simulink model "SecRwLtStFwdBkwdIsPosChk"  (R2024b)
settings: Solver=FixedStepDiscrete  StartTime=0.0  StopTime=10.0  FixedStep=0.01  RelTol=1e-3
undefined symbols (not defined in the file or in its folder): KeSMSuSecRwStFwdBkwdPosDelta_Val, KeSMSuSecRwStFwdBkwdPosTolr_Val
libraries: StIsPosChkLib x11, simulink x7
(part 1 of 2)
settings Model: Creator=sn2xws  LastModifiedBy=sn55gm
settings Model: ModifiedHistory=|
  | 2023.8.1 V2.0.0 CR421790 增加模式21-26
  | 2023.9.14 V2.1.0 Bug 540886 修改亲密模式判断到位的条件为10ms周期计算
  | 2023.11.16 V2.3.0 Issue 566045 全躺，vip，腿托打开增加前后位置
  | 2024.7.8 V3.0.0 557模式流程V1.9
  | 2024.8.15 V3.0.1 智享模式需要计算目标位置，不能直接判断到位置，posalready赋值0
  | 2024.9.4 V3.0.2 增加模式Md56，注释不使用的模式
  | 2024.9.18 V3.0.3 Md27 被误注释恢复
  | 2024.10.28 V3.0.4 Md56Calib标签名使用错误导致Md56前后目标位置为0
  | 2024.12.17 V3.0.5 Md57 Md58 报失败问题
  | 25.7.1 V3.13.0 新增Md61Md62
settings SolverCC: AlgebraicLoopSolver=TrustRegion
settings DataIOCC: SaveFormat=StructureWithTime  ReturnWorkspaceOutputs=off
settings OptimizationCC: DefaultParameterBehavior=Inlined  EnhancedBackFolding=on  PassReuseOutputArgsAs=Individual arguments  ZeroExternalMemoryAtStartup=off  ZeroInternalMemoryAtStartup=off  OptimizeBlockOrder=speed  DifferentSizesBufferReuse=on  OptimizationCustomize=off  EfficientTunableParamExpr=on
settings DebuggingCC: ParameterTunabilityLossMsg=error  UnconnectedInputMsg=warning  UnconnectedOutputMsg=warning  UnconnectedLineMsg=warning  ArithmeticOperatorsInVariantConditions=warning
settings ModelReferenceCC: EnableRefExpFcnMdlSchedulingChecks=on  ModelReferenceNumInstancesAllowed=Single
settings SFSimCC: MATLABDynamicMemAlloc=off  CustomCodeUndefinedFunction=UseInterfaceOnly
settings RTWCC: Description=AUTOSAR  SystemTargetFile=autosar.tlc  GenCodeOnly=on  TemplateMakefile=ert_default_tmf  GenerateReport=on  IncludeHyperlinkInReport=on  LaunchReport=on  DataTypeReplacement=CDataTypesFixedWidth  GenerateTraceInfo=on  GenerateTraceReport=on  GenerateTraceReportSl=on  GenerateTraceReportSf=on  GenerateTraceReportEml=on  GenerateCodeMetricsReport=on  GPUComputeCapability=3.5
settings CodeAppCC: ForceParamTrailComments=on  IgnoreCustomStorageClasses=off  OperatorAnnotations=on  SimulinkDataObjDesc=on  SFDataObjDesc=on  InsertBlockDesc=on
settings STFCustomTargetCC: TargetLangStandard=C99 (ISO)  MultiwordLength=256  ParMdlRefBuildCompliant=on  CompOptLevelCompliant=on  IncludeMdlTerminateFcn=off  CombineOutputUpdateFcns=on  SuppressErrorStatus=on  ERTCustomFileBanners=on  SupportNonFinite=off  SupportComplex=off  SupportContinuousTime=off  SupportNonInlinedSFcns=off  RemoveResetFunc=on  MATLABClassNameForMDSCustomization=Simulink.SoftwareTarget.ERTCustomization  AutosarCompliant=on  UseToolchainInfoCompliant=on  LookupTableObjectStructAxisOrder=2,1,3,4,...  LUTObjectStructOrderEvenSpacing=Size,Table,Breakpoints  SystemTargetFile=autosar.tlc
settings ERTTargetCC: TargetLangStandard=C99 (ISO)  ConcurrentExecutionCompliant=off  IncludeMdlTerminateFcn=off  SuppressErrorStatus=on  SupportNonFinite=off  SupportComplex=off  ModelStepFunctionPrototypeControlCompliant=off  CPPClassGenCompliant=off  AutosarCompliant=on  LookupTableObjectStructAxisOrder=2,1,3,4,...  LUTObjectStructOrderEvenSpacing=Size,Table,Breakpoints  ERTCustomFileTemplate=example_file_process.tlc  ERTFilePackagingFormat=Compact  BooleanTrueId=TRUE  BooleanFalseId=FALSE  DynamicArrayContainerType=coder::array

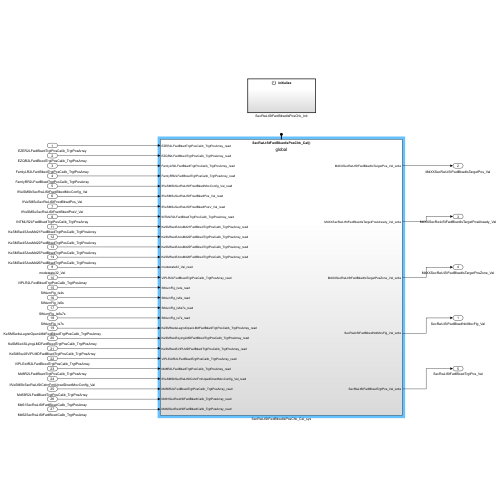
[thumbnail: Simulink's stored preview of the top-level diagram]
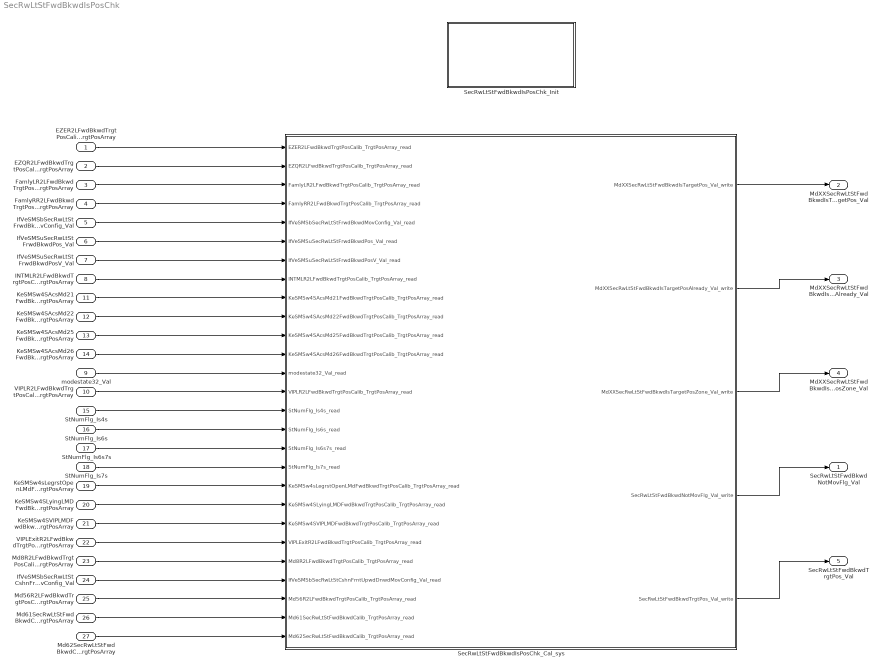
== system SecRwLtStFwdBkwdIsPosChk ==
  EZER2LFwdBkwdTrgtPosCalib_TrgtPosArray : Inport  Description=|  OutDataTypeStr=uint16  PortDimensions=3
      | 0:Pos
      | 1:Max
      | 2:Min
  EZQR2LFwdBkwdTrgtPosCalib_TrgtPosArray : Inport  Description=|  Port=2  OutDataTypeStr=uint16  PortDimensions=3
      | 0:Pos
      | 1:Max
      | 2:Min
  FamlyLR2LFwdBkwdTrgtPosCalib_TrgtPosArray : Inport  Description=|  Port=3  OutDataTypeStr=uint16  PortDimensions=3
      | 0:Pos
      | 1:Max
      | 2:Min
  FamlyRR2LFwdBkwdTrgtPosCalib_TrgtPosArray : Inport  Description=|  Port=4  OutDataTypeStr=uint16  PortDimensions=3
      | 0:Pos
      | 1:Max
      | 2:Min
  IfVeSMSbSecRwLtStFrwdBkwdMovConfig_Val : Inport  Port=5  OutDataTypeStr=boolean  PortDimensions=1
  IfVeSMSuSecRwLtStFrwdBkwdPos_Val : Inport  Port=6  OutDataTypeStr=uint16  PortDimensions=1
  IfVeSMSuSecRwLtStFrwdBkwdPosV_Val : Inport  Port=7  OutDataTypeStr=boolean  PortDimensions=1
  INTMLR2LFwdBkwdTrgtPosCalib_TrgtPosArray : Inport  Description=|  Port=8  OutDataTypeStr=uint16  PortDimensions=3
      | 0:Pos
      | 1:Max
      | 2:Min
  modestate32_Val : Inport  Port=9  OutDataTypeStr=uint32  PortDimensions=1
  VIPLR2LFwdBkwdTrgtPosCalib_TrgtPosArray : Inport  Description=|  Port=10  OutDataTypeStr=uint16  PortDimensions=3
      | 0:Pos
      | 1:Max
      | 2:Min
  KeSMSw4SAcsMd21FwdBkwdTrgtPosCalib_TrgtPosArray : Inport  Description=|  Port=11  OutDataTypeStr=uint16  PortDimensions=3
      | 0:Pos
      | 1:Max
      | 2:Min
  KeSMSw4SAcsMd22FwdBkwdTrgtPosCalib_TrgtPosArray : Inport  Description=|  Port=12  OutDataTypeStr=uint16  PortDimensions=3
      | 0:Pos
      | 1:Max
      | 2:Min
  KeSMSw4SAcsMd25FwdBkwdTrgtPosCalib_TrgtPosArray : Inport  Description=|  Port=13  OutDataTypeStr=uint16  PortDimensions=3
      | 0:Pos
      | 1:Max
      | 2:Min
  KeSMSw4SAcsMd26FwdBkwdTrgtPosCalib_TrgtPosArray : Inport  Description=|  Port=14  OutDataTypeStr=uint16  PortDimensions=3
      | 0:Pos
      | 1:Max
      | 2:Min
  StNumFlg_Is4s : Inport  Port=15  OutDataTypeStr=boolean  PortDimensions=1
  StNumFlg_Is6s : Inport  Port=16  OutDataTypeStr=boolean  PortDimensions=1
  StNumFlg_Is6s7s : Inport  Port=17  OutDataTypeStr=boolean  PortDimensions=1
  StNumFlg_Is7s : Inport  Port=18  OutDataTypeStr=boolean  PortDimensions=1
  KeSMSw4sLegrstOpenLMdFwdBkwdTrgtPosCalib_TrgtPosArray : Inport  Description=|  Port=19  OutDataTypeStr=uint16  PortDimensions=3
      | 0:Pos
      | 1:Max
      | 2:Min
  KeSMSw4SLyingLMDFwdBkwdTrgtPosCalib_TrgtPosArray : Inport  Description=|  Port=20  OutDataTypeStr=uint16  PortDimensions=3
      | 0:Pos
      | 1:Max
      | 2:Min
  KeSMSw4SVIPLMDFwdBkwdTrgtPosCalib_TrgtPosArray : Inport  Description=|  Port=21  OutDataTypeStr=uint16  PortDimensions=3
      | 0:Pos
      | 1:Max
      | 2:Min
  VIPLExitR2LFwdBkwdTrgtPosCalib_TrgtPosArray : Inport  Description=|  Port=22  OutDataTypeStr=uint16  PortDimensions=3
      | 0:Pos
      | 1:Max
      | 2:Min
  Md8R2LFwdBkwdTrgtPosCalib_TrgtPosArray : Inport  Description=|  Port=23  OutDataTypeStr=uint16  PortDimensions=3
      | 0:Pos
      | 1:Max
      | 2:Min
  IfVeSMSbSecRwLtStCshnFrntUpwdDnwdMovConfig_Val : Inport  Port=24  OutDataTypeStr=boolean  PortDimensions=1
  Md56R2LFwdBkwdTrgtPosCalib_TrgtPosArray : Inport  Description=|  Port=25  OutDataTypeStr=uint16  PortDimensions=3
      | 0:Pos
      | 1:Max
      | 2:Min
  Md61SecRwLtStFwdBkwdCalib_TrgtPosArray : Inport  Description=|  Port=26  OutDataTypeStr=uint16  PortDimensions=3
      | 0:Pos
      | 1:Max
      | 2:Min
  Md62SecRwLtStFwdBkwdCalib_TrgtPosArray : Inport  Description=|  Port=27  OutDataTypeStr=uint16  PortDimensions=3
      | 0:Pos
      | 1:Max
      | 2:Min
  SecRwLtStFwdBkwdIsPosChk_Cal_sys : Subsystem
  SecRwLtStFwdBkwdIsPosChk_Init : Subsystem
  SecRwLtStFwdBkwdNotMovFlg_Val : Outport  OutDataTypeStr=boolean  PortDimensions=1  VectorParamsAs1DForOutWhenUnconnected=off
  MdXXSecRwLtStFwdBkwdIsTargetPos_Val : Outport  Port=2  OutDataTypeStr=uint32  PortDimensions=1  VectorParamsAs1DForOutWhenUnconnected=off
  MdXXSecRwLtStFwdBkwdIsTargetPosAlready_Val : Outport  Port=3  OutDataTypeStr=uint32  PortDimensions=1  VectorParamsAs1DForOutWhenUnconnected=off
  MdXXSecRwLtStFwdBkwdIsTargetPosZone_Val : Outport  Port=4  OutDataTypeStr=uint32  PortDimensions=1  VectorParamsAs1DForOutWhenUnconnected=off
  SecRwLtStFwdBkwdTrgtPos_Val : Outport  Port=5  OutDataTypeStr=uint16  PortDimensions=1  VectorParamsAs1DForOutWhenUnconnected=off
  wires:
  EZER2LFwdBkwdTrgtPosCalib_TrgtPosArray/1 -> SecRwLtStFwdBkwdIsPosChk_Cal_sys/1(EZER2LFwdBkwdTrgtPosCalib_TrgtPosArray_read)
  EZQR2LFwdBkwdTrgtPosCalib_TrgtPosArray/1 -> SecRwLtStFwdBkwdIsPosChk_Cal_sys/2(EZQR2LFwdBkwdTrgtPosCalib_TrgtPosArray_read)
  FamlyLR2LFwdBkwdTrgtPosCalib_TrgtPosArray/1 -> SecRwLtStFwdBkwdIsPosChk_Cal_sys/3(FamlyLR2LFwdBkwdTrgtPosCalib_TrgtPosArray_read)
  FamlyRR2LFwdBkwdTrgtPosCalib_TrgtPosArray/1 -> SecRwLtStFwdBkwdIsPosChk_Cal_sys/4(FamlyRR2LFwdBkwdTrgtPosCalib_TrgtPosArray_read)
  IfVeSMSbSecRwLtStFrwdBkwdMovConfig_Val/1 -> SecRwLtStFwdBkwdIsPosChk_Cal_sys/5(IfVeSMSbSecRwLtStFrwdBkwdMovConfig_Val_read)
  IfVeSMSuSecRwLtStFrwdBkwdPos_Val/1 -> SecRwLtStFwdBkwdIsPosChk_Cal_sys/6(IfVeSMSuSecRwLtStFrwdBkwdPos_Val_read)
  IfVeSMSuSecRwLtStFrwdBkwdPosV_Val/1 -> SecRwLtStFwdBkwdIsPosChk_Cal_sys/7(IfVeSMSuSecRwLtStFrwdBkwdPosV_Val_read)
  INTMLR2LFwdBkwdTrgtPosCalib_TrgtPosArray/1 -> SecRwLtStFwdBkwdIsPosChk_Cal_sys/8(INTMLR2LFwdBkwdTrgtPosCalib_TrgtPosArray_read)
  modestate32_Val/1 -> SecRwLtStFwdBkwdIsPosChk_Cal_sys/13(modestate32_Val_read)
  VIPLR2LFwdBkwdTrgtPosCalib_TrgtPosArray/1 -> SecRwLtStFwdBkwdIsPosChk_Cal_sys/14(VIPLR2LFwdBkwdTrgtPosCalib_TrgtPosArray_read)
  SecRwLtStFwdBkwdIsPosChk_Cal_sys/1(MdXXSecRwLtStFwdBkwdIsTargetPos_Val_write) -> MdXXSecRwLtStFwdBkwdIsTargetPos_Val/1
  SecRwLtStFwdBkwdIsPosChk_Cal_sys/2(MdXXSecRwLtStFwdBkwdIsTargetPosAlready_Val_write) -> MdXXSecRwLtStFwdBkwdIsTargetPosAlready_Val/1
  SecRwLtStFwdBkwdIsPosChk_Cal_sys/3(MdXXSecRwLtStFwdBkwdIsTargetPosZone_Val_write) -> MdXXSecRwLtStFwdBkwdIsTargetPosZone_Val/1
  SecRwLtStFwdBkwdIsPosChk_Cal_sys/4(SecRwLtStFwdBkwdNotMovFlg_Val_write) -> SecRwLtStFwdBkwdNotMovFlg_Val/1
  SecRwLtStFwdBkwdIsPosChk_Cal_sys/5(SecRwLtStFwdBkwdTrgtPos_Val_write) -> SecRwLtStFwdBkwdTrgtPos_Val/1
  KeSMSw4SAcsMd21FwdBkwdTrgtPosCalib_TrgtPosArray/1 -> SecRwLtStFwdBkwdIsPosChk_Cal_sys/9(KeSMSw4SAcsMd21FwdBkwdTrgtPosCalib_TrgtPosArray_read)
  KeSMSw4SAcsMd22FwdBkwdTrgtPosCalib_TrgtPosArray/1 -> SecRwLtStFwdBkwdIsPosChk_Cal_sys/10(KeSMSw4SAcsMd22FwdBkwdTrgtPosCalib_TrgtPosArray_read)
  KeSMSw4SAcsMd25FwdBkwdTrgtPosCalib_TrgtPosArray/1 -> SecRwLtStFwdBkwdIsPosChk_Cal_sys/11(KeSMSw4SAcsMd25FwdBkwdTrgtPosCalib_TrgtPosArray_read)
  KeSMSw4SAcsMd26FwdBkwdTrgtPosCalib_TrgtPosArray/1 -> SecRwLtStFwdBkwdIsPosChk_Cal_sys/12(KeSMSw4SAcsMd26FwdBkwdTrgtPosCalib_TrgtPosArray_read)
  StNumFlg_Is4s/1 -> SecRwLtStFwdBkwdIsPosChk_Cal_sys/15(StNumFlg_Is4s_read)
  StNumFlg_Is6s/1 -> SecRwLtStFwdBkwdIsPosChk_Cal_sys/16(StNumFlg_Is6s_read)
  StNumFlg_Is6s7s/1 -> SecRwLtStFwdBkwdIsPosChk_Cal_sys/17(StNumFlg_Is6s7s_read)
  StNumFlg_Is7s/1 -> SecRwLtStFwdBkwdIsPosChk_Cal_sys/18(StNumFlg_Is7s_read)
  KeSMSw4sLegrstOpenLMdFwdBkwdTrgtPosCalib_TrgtPosArray/1 -> SecRwLtStFwdBkwdIsPosChk_Cal_sys/19(KeSMSw4sLegrstOpenLMdFwdBkwdTrgtPosCalib_TrgtPosArray_read)
  KeSMSw4SLyingLMDFwdBkwdTrgtPosCalib_TrgtPosArray/1 -> SecRwLtStFwdBkwdIsPosChk_Cal_sys/20(KeSMSw4SLyingLMDFwdBkwdTrgtPosCalib_TrgtPosArray_read)
  KeSMSw4SVIPLMDFwdBkwdTrgtPosCalib_TrgtPosArray/1 -> SecRwLtStFwdBkwdIsPosChk_Cal_sys/21(KeSMSw4SVIPLMDFwdBkwdTrgtPosCalib_TrgtPosArray_read)
  VIPLExitR2LFwdBkwdTrgtPosCalib_TrgtPosArray/1 -> SecRwLtStFwdBkwdIsPosChk_Cal_sys/22(VIPLExitR2LFwdBkwdTrgtPosCalib_TrgtPosArray_read)
  Md8R2LFwdBkwdTrgtPosCalib_TrgtPosArray/1 -> SecRwLtStFwdBkwdIsPosChk_Cal_sys/23(Md8R2LFwdBkwdTrgtPosCalib_TrgtPosArray_read)
  IfVeSMSbSecRwLtStCshnFrntUpwdDnwdMovConfig_Val/1 -> SecRwLtStFwdBkwdIsPosChk_Cal_sys/24(IfVeSMSbSecRwLtStCshnFrntUpwdDnwdMovConfig_Val_read)
  Md56R2LFwdBkwdTrgtPosCalib_TrgtPosArray/1 -> SecRwLtStFwdBkwdIsPosChk_Cal_sys/25(Md56R2LFwdBkwdTrgtPosCalib_TrgtPosArray_read)
  Md61SecRwLtStFwdBkwdCalib_TrgtPosArray/1 -> SecRwLtStFwdBkwdIsPosChk_Cal_sys/26(Md61SecRwLtStFwdBkwdCalib_TrgtPosArray_read)
  Md62SecRwLtStFwdBkwdCalib_TrgtPosArray/1 -> SecRwLtStFwdBkwdIsPosChk_Cal_sys/27(Md62SecRwLtStFwdBkwdCalib_TrgtPosArray_read)

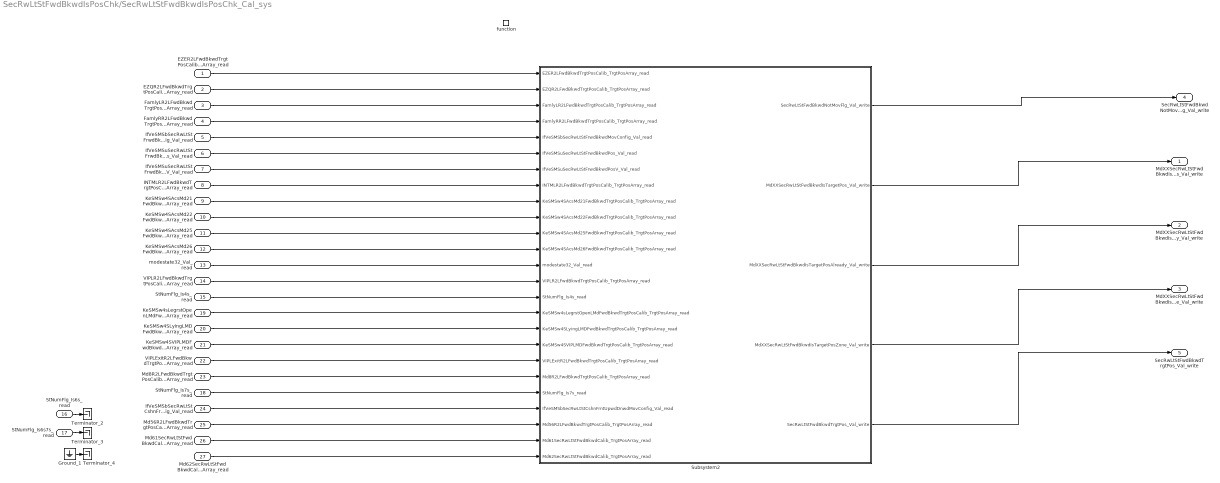
== system SecRwLtStFwdBkwdIsPosChk/SecRwLtStFwdBkwdIsPosChk_Cal_sys ==
  EZER2LFwdBkwdTrgtPosCalib_TrgtPosArray_read : Inport
  EZQR2LFwdBkwdTrgtPosCalib_TrgtPosArray_read : Inport  Port=2
  FamlyLR2LFwdBkwdTrgtPosCalib_TrgtPosArray_read : Inport  Port=3
  FamlyRR2LFwdBkwdTrgtPosCalib_TrgtPosArray_read : Inport  Port=4
  IfVeSMSbSecRwLtStFrwdBkwdMovConfig_Val_read : Inport  Port=5
  IfVeSMSuSecRwLtStFrwdBkwdPos_Val_read : Inport  Port=6
  IfVeSMSuSecRwLtStFrwdBkwdPosV_Val_read : Inport  Port=7
  INTMLR2LFwdBkwdTrgtPosCalib_TrgtPosArray_read : Inport  Port=8
  KeSMSw4SAcsMd21FwdBkwdTrgtPosCalib_TrgtPosArray_read : Inport  Port=9
  KeSMSw4SAcsMd22FwdBkwdTrgtPosCalib_TrgtPosArray_read : Inport  Port=10
  KeSMSw4SAcsMd25FwdBkwdTrgtPosCalib_TrgtPosArray_read : Inport  Port=11
  KeSMSw4SAcsMd26FwdBkwdTrgtPosCalib_TrgtPosArray_read : Inport  Port=12
  modestate32_Val_read : Inport  Port=13
  VIPLR2LFwdBkwdTrgtPosCalib_TrgtPosArray_read : Inport  Port=14
  StNumFlg_Is4s_read : Inport  Port=15
  StNumFlg_Is6s_read : Inport  Port=16
  StNumFlg_Is6s7s_read : Inport  Port=17
  StNumFlg_Is7s_read : Inport  Port=18
  KeSMSw4sLegrstOpenLMdFwdBkwdTrgtPosCalib_TrgtPosArray_read : Inport  Port=19
  KeSMSw4SLyingLMDFwdBkwdTrgtPosCalib_TrgtPosArray_read : Inport  Port=20
  KeSMSw4SVIPLMDFwdBkwdTrgtPosCalib_TrgtPosArray_read : Inport  Port=21
  VIPLExitR2LFwdBkwdTrgtPosCalib_TrgtPosArray_read : Inport  Port=22
  Md8R2LFwdBkwdTrgtPosCalib_TrgtPosArray_read : Inport  Port=23
  IfVeSMSbSecRwLtStCshnFrntUpwdDnwdMovConfig_Val_read : Inport  Port=24
  Md56R2LFwdBkwdTrgtPosCalib_TrgtPosArray_read : Inport  Port=25
  Md61SecRwLtStFwdBkwdCalib_TrgtPosArray_read : Inport  Port=26
  Md62SecRwLtStFwdBkwdCalib_TrgtPosArray_read : Inport  Port=27
  function : TriggerPort  TriggerType=function-call  IsSimulinkFunction=on  FunctionName=SecRwLtStFwdBkwdIsPosChk_Cal  VariantControl=(inherit)
  Ground_1 : Ground
  Subsystem2 : Subsystem
  Terminator_2 : Terminator
  Terminator_3 : Terminator
  Terminator_4 : Terminator
  MdXXSecRwLtStFwdBkwdIsTargetPos_Val_write : Outport  VectorParamsAs1DForOutWhenUnconnected=off
      settings: EnsureOutportIsVirtual=on
  MdXXSecRwLtStFwdBkwdIsTargetPosAlready_Val_write : Outport  Port=2  VectorParamsAs1DForOutWhenUnconnected=off
      settings: EnsureOutportIsVirtual=on
  MdXXSecRwLtStFwdBkwdIsTargetPosZone_Val_write : Outport  Port=3  VectorParamsAs1DForOutWhenUnconnected=off
      settings: EnsureOutportIsVirtual=on
  SecRwLtStFwdBkwdNotMovFlg_Val_write : Outport  Port=4  VectorParamsAs1DForOutWhenUnconnected=off
      settings: EnsureOutportIsVirtual=on
  SecRwLtStFwdBkwdTrgtPos_Val_write : Outport  Port=5  VectorParamsAs1DForOutWhenUnconnected=off
      settings: EnsureOutportIsVirtual=on
  wires:
  Subsystem2/1(SecRwLtStFwdBkwdNotMovFlg_Val_write) -> SecRwLtStFwdBkwdNotMovFlg_Val_write/1
  Subsystem2/2(MdXXSecRwLtStFwdBkwdIsTargetPos_Val_write) -> MdXXSecRwLtStFwdBkwdIsTargetPos_Val_write/1
  Subsystem2/3(MdXXSecRwLtStFwdBkwdIsTargetPosAlready_Val_write) -> MdXXSecRwLtStFwdBkwdIsTargetPosAlready_Val_write/1
  Subsystem2/4(MdXXSecRwLtStFwdBkwdIsTargetPosZone_Val_write) -> MdXXSecRwLtStFwdBkwdIsTargetPosZone_Val_write/1
  Subsystem2/5(SecRwLtStFwdBkwdTrgtPos_Val_write) -> SecRwLtStFwdBkwdTrgtPos_Val_write/1
  EZER2LFwdBkwdTrgtPosCalib_TrgtPosArray_read/1 -> Subsystem2/1(EZER2LFwdBkwdTrgtPosCalib_TrgtPosArray_read)
  EZQR2LFwdBkwdTrgtPosCalib_TrgtPosArray_read/1 -> Subsystem2/2(EZQR2LFwdBkwdTrgtPosCalib_TrgtPosArray_read)
  FamlyLR2LFwdBkwdTrgtPosCalib_TrgtPosArray_read/1 -> Subsystem2/3(FamlyLR2LFwdBkwdTrgtPosCalib_TrgtPosArray_read)
  FamlyRR2LFwdBkwdTrgtPosCalib_TrgtPosArray_read/1 -> Subsystem2/4(FamlyRR2LFwdBkwdTrgtPosCalib_TrgtPosArray_read)
  IfVeSMSbSecRwLtStFrwdBkwdMovConfig_Val_read/1 -> Subsystem2/5(IfVeSMSbSecRwLtStFrwdBkwdMovConfig_Val_read)
  IfVeSMSuSecRwLtStFrwdBkwdPos_Val_read/1 -> Subsystem2/6(IfVeSMSuSecRwLtStFrwdBkwdPos_Val_read)
  IfVeSMSuSecRwLtStFrwdBkwdPosV_Val_read/1 -> Subsystem2/7(IfVeSMSuSecRwLtStFrwdBkwdPosV_Val_read)
  INTMLR2LFwdBkwdTrgtPosCalib_TrgtPosArray_read/1 -> Subsystem2/8(INTMLR2LFwdBkwdTrgtPosCalib_TrgtPosArray_read)
  KeSMSw4SAcsMd21FwdBkwdTrgtPosCalib_TrgtPosArray_read/1 -> Subsystem2/9(KeSMSw4SAcsMd21FwdBkwdTrgtPosCalib_TrgtPosArray_read)
  KeSMSw4SAcsMd22FwdBkwdTrgtPosCalib_TrgtPosArray_read/1 -> Subsystem2/10(KeSMSw4SAcsMd22FwdBkwdTrgtPosCalib_TrgtPosArray_read)
  KeSMSw4SAcsMd25FwdBkwdTrgtPosCalib_TrgtPosArray_read/1 -> Subsystem2/11(KeSMSw4SAcsMd25FwdBkwdTrgtPosCalib_TrgtPosArray_read)
  KeSMSw4SAcsMd26FwdBkwdTrgtPosCalib_TrgtPosArray_read/1 -> Subsystem2/12(KeSMSw4SAcsMd26FwdBkwdTrgtPosCalib_TrgtPosArray_read)
  modestate32_Val_read/1 -> Subsystem2/13(modestate32_Val_read)
  VIPLR2LFwdBkwdTrgtPosCalib_TrgtPosArray_read/1 -> Subsystem2/14(VIPLR2LFwdBkwdTrgtPosCalib_TrgtPosArray_read)
  StNumFlg_Is4s_read/1 -> Subsystem2/15(StNumFlg_Is4s_read)
  StNumFlg_Is6s_read/1 -> Terminator_2/1
  StNumFlg_Is6s7s_read/1 -> Terminator_3/1
  KeSMSw4sLegrstOpenLMdFwdBkwdTrgtPosCalib_TrgtPosArray_read/1 -> Subsystem2/16(KeSMSw4sLegrstOpenLMdFwdBkwdTrgtPosCalib_TrgtPosArray_read)
  KeSMSw4SLyingLMDFwdBkwdTrgtPosCalib_TrgtPosArray_read/1 -> Subsystem2/17(KeSMSw4SLyingLMDFwdBkwdTrgtPosCalib_TrgtPosArray_read)
  KeSMSw4SVIPLMDFwdBkwdTrgtPosCalib_TrgtPosArray_read/1 -> Subsystem2/18(KeSMSw4SVIPLMDFwdBkwdTrgtPosCalib_TrgtPosArray_read)
  VIPLExitR2LFwdBkwdTrgtPosCalib_TrgtPosArray_read/1 -> Subsystem2/19(VIPLExitR2LFwdBkwdTrgtPosCalib_TrgtPosArray_read)
  Md8R2LFwdBkwdTrgtPosCalib_TrgtPosArray_read/1 -> Subsystem2/20(Md8R2LFwdBkwdTrgtPosCalib_TrgtPosArray_read)
  StNumFlg_Is7s_read/1 -> Subsystem2/21(StNumFlg_Is7s_read)
  IfVeSMSbSecRwLtStCshnFrntUpwdDnwdMovConfig_Val_read/1 -> Subsystem2/22(IfVeSMSbSecRwLtStCshnFrntUpwdDnwdMovConfig_Val_read)
  Ground_1/1 -> Terminator_4/1
  Md56R2LFwdBkwdTrgtPosCalib_TrgtPosArray_read/1 -> Subsystem2/23(Md56R2LFwdBkwdTrgtPosCalib_TrgtPosArray_read)
  Md61SecRwLtStFwdBkwdCalib_TrgtPosArray_read/1 -> Subsystem2/24(Md61SecRwLtStFwdBkwdCalib_TrgtPosArray_read)
  Md62SecRwLtStFwdBkwdCalib_TrgtPosArray_read/1 -> Subsystem2/25(Md62SecRwLtStFwdBkwdCalib_TrgtPosArray_read)

== system SecRwLtStFwdBkwdIsPosChk/SecRwLtStFwdBkwdIsPosChk_Init ==
  note: Added blocks
  note: Added blocks
  Event Listener : EventListener  EventName=reset
  PA_KeSMSuSecRwStFwdBkwdPosDelta_Val : Constant  Value=KeSMSuSecRwStFwdBkwdPosDelta_Val
  PA_KeSMSuSecRwStFwdBkwdPosTolr_Val : Constant  Value=KeSMSuSecRwStFwdBkwdPosTolr_Val
  Terminator_1 : Terminator
  Terminator_2 : Terminator
  wires:
  PA_KeSMSuSecRwStFwdBkwdPosDelta_Val/1 -> Terminator_1/1
  PA_KeSMSuSecRwStFwdBkwdPosTolr_Val/1 -> Terminator_2/1

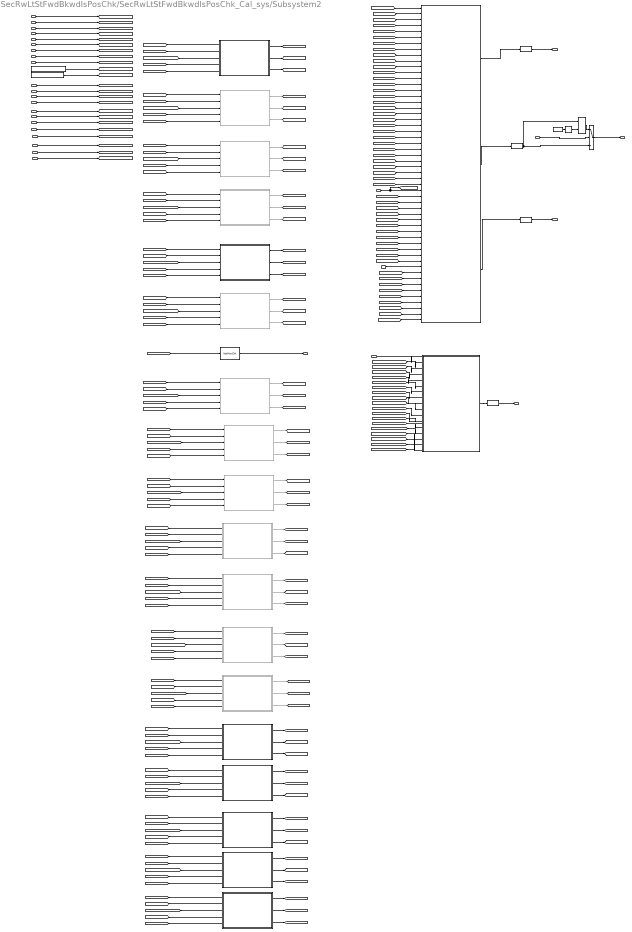
== system SecRwLtStFwdBkwdIsPosChk/SecRwLtStFwdBkwdIsPosChk_Cal_sys/Subsystem2 ==
  note: Issue 566045 全躺，vip，腿托打开增加前后位置
  note: 2023.9.14 V2.1.0 Bug 540886 修改亲密模式判断到位的条件为10ms周期计算
  note: 2023.8.1 V2.0.0 CR421790 增加模式21-26
  EZER2LFwdBkwdTrgtPosCalib_TrgtPosArray_read : Inport
  EZQR2LFwdBkwdTrgtPosCalib_TrgtPosArray_read : Inport  Port=2
  FamlyLR2LFwdBkwdTrgtPosCalib_TrgtPosArray_read : Inport  Port=3
  FamlyRR2LFwdBkwdTrgtPosCalib_TrgtPosArray_read : Inport  Port=4
  IfVeSMSbSecRwLtStFrwdBkwdMovConfig_Val_read : Inport  Port=5
  IfVeSMSuSecRwLtStFrwdBkwdPos_Val_read : Inport  Port=6
  IfVeSMSuSecRwLtStFrwdBkwdPosV_Val_read : Inport  Port=7
  INTMLR2LFwdBkwdTrgtPosCalib_TrgtPosArray_read : Inport  Port=8
  KeSMSw4SAcsMd21FwdBkwdTrgtPosCalib_TrgtPosArray_read : Inport  Port=9
  KeSMSw4SAcsMd22FwdBkwdTrgtPosCalib_TrgtPosArray_read : Inport  Port=10
  KeSMSw4SAcsMd25FwdBkwdTrgtPosCalib_TrgtPosArray_read : Inport  Port=11
  KeSMSw4SAcsMd26FwdBkwdTrgtPosCalib_TrgtPosArray_read : Inport  Port=12
  modestate32_Val_read : Inport  Port=13
  VIPLR2LFwdBkwdTrgtPosCalib_TrgtPosArray_read : Inport  Port=14
  StNumFlg_Is4s_read : Inport  Port=15
  KeSMSw4sLegrstOpenLMdFwdBkwdTrgtPosCalib_TrgtPosArray_read : Inport  Port=16
  KeSMSw4SLyingLMDFwdBkwdTrgtPosCalib_TrgtPosArray_read : Inport  Port=17
  KeSMSw4SVIPLMDFwdBkwdTrgtPosCalib_TrgtPosArray_read : Inport  Port=18
  VIPLExitR2LFwdBkwdTrgtPosCalib_TrgtPosArray_read : Inport  Port=19
  Md8R2LFwdBkwdTrgtPosCalib_TrgtPosArray_read : Inport  Port=20
  StNumFlg_Is7s_read : Inport  Port=21
  IfVeSMSbSecRwLtStCshnFrntUpwdDnwdMovConfig_Val_read : Inport  Port=22
  Md56R2LFwdBkwdTrgtPosCalib_TrgtPosArray_read : Inport  Port=23
  Md61SecRwLtStFwdBkwdCalib_TrgtPosArray_read : Inport  Port=24
  Md62SecRwLtStFwdBkwdCalib_TrgtPosArray_read : Inport  Port=25
  Bitwise Operator : simulink/Logic and Bit Operations/Bitwise Operator  logicop=AND  UseBitMask=off  NumInputPorts=2  BitMask=bin2dec('11011001')  BitMaskRealWorld=Stored Integer
  Bitwise Operator1 : simulink/Logic and Bit Operations/Bitwise Operator  logicop=NOT  UseBitMask=off  BitMask=bin2dec('11011001')  BitMaskRealWorld=Stored Integer
  Constant : Constant  Value=512  OutDataTypeStr=uint32
  Data Type Conversion{,1..3} (4 alike) : DataTypeConversion  SaturateOnIntegerOverflow=off  RndMeth=Floor
  NotMovChk : StIsPosChkLib/NotMovChk  SystemSampleTime=-1  VariantActivationTime=update diagram  AllowFlexibleInterface=on  Latency=0  AutoFrameSizeCalculation=off
  PA_KeSMSuSecRwStFwdBkwdPosDelta_Val : Constant  Value=KeSMSuSecRwStFwdBkwdPosDelta_Val
  PA_KeSMSuSecRwStFwdBkwdPosTolr_Val : Constant  Value=KeSMSuSecRwStFwdBkwdPosTolr_Val
  Subsystem : Subsystem
  Subsystem1 : Subsystem
  Subsystem10 : Subsystem  Commented=on
  Subsystem11 : Subsystem  Commented=on
  Subsystem12 : Subsystem  Commented=on
  Subsystem13 : Subsystem  Commented=on
  Subsystem14 : Subsystem  Commented=on
  Subsystem15 : Subsystem
  Subsystem16 : Subsystem
  Subsystem17 : Subsystem
  Subsystem18 : Subsystem
  Subsystem19 : Subsystem
  Subsystem2 : Subsystem
  Subsystem3 : Subsystem  Commented=on
  Subsystem4 : Subsystem  Commented=on
  Subsystem5 : Subsystem  Commented=on
  Subsystem6 : Subsystem
  Subsystem7 : Subsystem  Commented=on
  Subsystem8 : Subsystem  Commented=on
  Subsystem9 : Subsystem  Commented=on
  Switch : Switch  Criteria=u2 > Threshold  SaturateOnIntegerOverflow=off  InputSameDT=off
  SecRwLtStFwdBkwdNotMovFlg_Val_write : Outport  VectorParamsAs1DForOutWhenUnconnected=off
      settings: EnsureOutportIsVirtual=on
  MdXXSecRwLtStFwdBkwdIsTargetPos_Val_write : Outport  Port=2  VectorParamsAs1DForOutWhenUnconnected=off
      settings: EnsureOutportIsVirtual=on
  MdXXSecRwLtStFwdBkwdIsTargetPosAlready_Val_write : Outport  Port=3  VectorParamsAs1DForOutWhenUnconnected=off
      settings: EnsureOutportIsVirtual=on
  MdXXSecRwLtStFwdBkwdIsTargetPosZone_Val_write : Outport  Port=4  VectorParamsAs1DForOutWhenUnconnected=off
      settings: EnsureOutportIsVirtual=on
  SecRwLtStFwdBkwdTrgtPos_Val_write : Outport  Port=5  VectorParamsAs1DForOutWhenUnconnected=off
      settings: EnsureOutportIsVirtual=on
  wires:
  Subsystem7/1(IsPos) -> [INTMLIsTargetPos]
  VIPLR2LFwdBkwdTrgtPosCalib_TrgtPosArray_read/1 -> [VIPLCalib]
  IfVeSMSbSecRwLtStFrwdBkwdMovConfig_Val_read/1 -> [MovConfig]
  Subsystem3/2(IsPosZone) -> [EZQIsTargetPosZone]
  Subsystem2/3(IsPosAlready) -> [EZEIsTargetPosAlready]
  Subsystem5/2(IsPosZone) -> [FamlyRIsTargetPosZone]
  PA_KeSMSuSecRwStFwdBkwdPosDelta_Val/1 -> [PosDelta]
  [PosDelta] -> Subsystem3/4(Delta)
  EZQR2LFwdBkwdTrgtPosCalib_TrgtPosArray_read/1 -> [EZQCalib]
  [PosTolr] -> Subsystem6/5(Tolr)
  Subsystem4/3(IsPosAlready) -> [FamlyLIsTargetPosAlready]
  IfVeSMSuSecRwLtStFrwdBkwdPos_Val_read/1 -> [Pos]
  INTMLR2LFwdBkwdTrgtPosCalib_TrgtPosArray_read/1 -> [INTMLCalib]
  [FamlyRCalib] -> Subsystem5/3(CalibArray)
  Subsystem7/3(IsPosAlready) -> [INTMLIsTargetPosAlready]
  FamlyLR2LFwdBkwdTrgtPosCalib_TrgtPosArray_read/1 -> [FamlyLCalib]
  PA_KeSMSuSecRwStFwdBkwdPosTolr_Val/1 -> [PosTolr]
  [EZEIsTargetPos] -> Subsystem1/2(EZEIsTargetPos)
  [EZECalib] -> Subsystem2/3(CalibArray)
  [PosTolr] -> Subsystem5/5(Tolr)
  [EZEIsTargetPosZone] -> Subsystem1/14(EZEIsTargetPosZone)
  [MovConfig] -> Subsystem1/1(MovConfig)
  [PosDelta] -> Subsystem4/4(Delta)
  Subsystem6/3(IsPosAlready) -> [VIPLIsTargetPosAlready]
  Subsystem6/1(IsPos) -> [VIPLIsTargetPos]
  [VIPLIsTargetPosZone] -> Subsystem1/18(VIPLIsTargetPosZone)
  [PosTolr] -> Subsystem2/5(Tolr)
  Subsystem2/1(IsPos) -> [EZEIsTargetPos]
  [FamlyRIsTargetPosAlready] -> Subsystem1/11(FamlyRIsTargetPosAlready)
  Subsystem6/2(IsPosZone) -> [VIPLIsTargetPosZone]
  [PosV] -> Subsystem2/1(PosV)
  [PosTolr] -> Subsystem7/5(Tolr)
  [Pos] -> Subsystem2/2(Pos)
  [PosTolr] -> Subsystem4/5(Tolr)
  [FamlyLIsTargetPosAlready] -> Subsystem1/10(FamlyLIsTargetPosAlready)
  [PosDelta] -> Subsystem2/4(Delta)
  [PosV] -> Subsystem5/1(PosV)
  [Pos] -> NotMovChk/1
  Subsystem7/2(IsPosZone) -> [INTMLIsTargetPosZone]
  NotMovChk/1 -> SecRwLtStFwdBkwdNotMovFlg_Val_write/1
  Subsystem1/1(IsTargetPos) -> Data Type Conversion1/1
  Subsystem3/3(IsPosAlready) -> [EZQIsTargetPosAlready]
  FamlyRR2LFwdBkwdTrgtPosCalib_TrgtPosArray_read/1 -> [FamlyRCalib]
  [Pos] -> Subsystem4/2(Pos)
  [PosDelta] -> Subsystem5/4(Delta)
  [VIPLCalib] -> Subsystem/6(VIPLCalib)
  Subsystem4/2(IsPosZone) -> [FamlyLIsTargetPosZone]
  [Pos] -> Subsystem3/2(Pos)
  [EZQCalib] -> Subsystem3/3(CalibArray)
  [EZQCalib] -> Subsystem/3(EZQCalib)
  [PosV] -> Subsystem3/1(PosV)
  [FamlyRCalib] -> Subsystem/5(FamlyRCalib)
  Subsystem/1(TrgtPos) -> Data Type Conversion/1
  Subsystem2/2(IsPosZone) -> [EZEIsTargetPosZone]
  [PosTolr] -> Subsystem3/5(Tolr)
  Subsystem3/1(IsPos) -> [EZQIsTargetPos]
  [PosDelta] -> Subsystem7/4(Delta)
  IfVeSMSuSecRwLtStFrwdBkwdPosV_Val_read/1 -> [PosV]
  [VIPLIsTargetPos] -> Subsystem1/6(VIPLIsTargetPos)
  [EZQIsTargetPos] -> Subsystem1/3(EZQIsTargetPos)
  modestate32_Val_read/1 -> Subsystem/1(modestate32_Val_read)
  [PosV] -> Subsystem6/1(PosV)
  [VIPLIsTargetPosAlready] -> Subsystem1/12(VIPLIsTargetPosAlready)
  [PosV] -> Subsystem7/1(PosV)
  [EZEIsTargetPosAlready] -> Subsystem1/8(EZEIsTargetPosAlready)
  Data Type Conversion1/1 -> MdXXSecRwLtStFwdBkwdIsTargetPos_Val_write/1
  [EZECalib] -> Subsystem/2(EZECalib)
  [FamlyLCalib] -> Subsystem4/3(CalibArray)
  [FamlyLCalib] -> Subsystem/4(FamlyLCalib)
  [EZQIsTargetPosZone] -> Subsystem1/15(EZQIsTargetPosZone)
  [INTMLCalib] -> Subsystem7/3(CalibArray)
  [FamlyRIsTargetPos] -> Subsystem1/5(FamlyRIsTargetPos)
  EZER2LFwdBkwdTrgtPosCalib_TrgtPosArray_read/1 -> [EZECalib]
  Data Type Conversion3/1 -> MdXXSecRwLtStFwdBkwdIsTargetPosZone_Val_write/1
  Subsystem1/2(IsTargetPosAlready) -> Data Type Conversion2/1
  [Pos] -> Subsystem6/2(Pos)
  [FamlyLIsTargetPosZone] -> Subsystem1/16(FamlyLIsTargetPosZone)
  Subsystem4/1(IsPos) -> [FamlyLIsTargetPos]
  Subsystem5/1(IsPos) -> [FamlyRIsTargetPos]
  [VIPLCalib] -> Subsystem6/3(CalibArray)
  [PosV] -> Subsystem4/1(PosV)
  Subsystem1/3(IsTargetPosZone) -> Data Type Conversion3/1
  [FamlyLIsTargetPos] -> Subsystem1/4(FamlyLIsTargetPos)
  [Pos] -> Subsystem5/2(Pos)
  [FamlyRIsTargetPosZone] -> Subsystem1/17(FamlyRIsTargetPosZone)
  [INTMLCalib] -> Subsystem/7(INTMLCalib)
  [PosDelta] -> Subsystem6/4(Delta)
  [EZQIsTargetPosAlready] -> Subsystem1/9(EZQIsTargetPosAlready)
  [INTMLIsTargetPosZone] -> Subsystem1/19(INTMLIsTargetPosZone)
  Data Type Conversion/1 -> SecRwLtStFwdBkwdTrgtPos_Val_write/1
  [INTMLIsTargetPos] -> Subsystem1/7(INTMLIsTargetPos)
  Subsystem5/3(IsPosAlready) -> [FamlyRIsTargetPosAlready]
  [INTMLIsTargetPosAlready] -> Subsystem1/13(INTMLIsTargetPosAlready)
  [Pos] -> Subsystem7/2(Pos)
  KeSMSw4SAcsMd21FwdBkwdTrgtPosCalib_TrgtPosArray_read/1 -> [MD21Calib]
  KeSMSw4SAcsMd22FwdBkwdTrgtPosCalib_TrgtPosArray_read/1 -> [MD22Calib]
  KeSMSw4SAcsMd25FwdBkwdTrgtPosCalib_TrgtPosArray_read/1 -> [MD25Calib]
  KeSMSw4SAcsMd26FwdBkwdTrgtPosCalib_TrgtPosArray_read/1 -> [MD26Calib]
  [Pos] -> Subsystem8/2(Pos)
  [MD21Calib] -> Subsystem8/3(CalibArray)
  [PosV] -> Subsystem8/1(PosV)
  [PosDelta] -> Subsystem8/4(Delta)
  Subsystem8/2(IsPosZone) -> [Md21IsTargetPosZone]
  [PosTolr] -> Subsystem8/5(Tolr)
  Subsystem8/3(IsPosAlready) -> [Md21IsTargetPosAlready]
  Subsystem8/1(IsPos) -> [Md21IsTargetPos]
  Subsystem9/1(IsPos) -> [Md26IsTargetPos]
  Subsystem9/3(IsPosAlready) -> [Md26IsTargetPosAlready]
  [PosTolr] -> Subsystem9/5(Tolr)
  Subsystem9/2(IsPosZone) -> [Md26IsTargetPosZone]
  [PosDelta] -> Subsystem9/4(Delta)
  [PosV] -> Subsystem9/1(PosV)
  [MD26Calib] -> Subsystem9/3(CalibArray)
  [Pos] -> Subsystem9/2(Pos)
  [Pos] -> Subsystem10/2(Pos)
  [MD22Calib] -> Subsystem10/3(CalibArray)
  [PosV] -> Subsystem10/1(PosV)
  [PosDelta] -> Subsystem10/4(Delta)
  Subsystem10/2(IsPosZone) -> [Md22IsTargetPosZone]
  [PosTolr] -> Subsystem10/5(Tolr)
  Subsystem10/3(IsPosAlready) -> [Md22IsTargetPosAlready]
  Subsystem10/1(IsPos) -> [Md22IsTargetPos]
  Subsystem11/1(IsPos) -> [Md25IsTargetPos]
  Subsystem11/3(IsPosAlready) -> [Md25IsTargetPosAlready]
  [PosTolr] -> Subsystem11/5(Tolr)
  Subsystem11/2(IsPosZone) -> [Md25IsTargetPosZone]
  [PosDelta] -> Subsystem11/4(Delta)
  [PosV] -> Subsystem11/1(PosV)
  [MD25Calib] -> Subsystem11/3(CalibArray)
  [Pos] -> Subsystem11/2(Pos)
  [MD21Calib] -> Subsystem/8(Md21Calib)
  [MD22Calib] -> Subsystem/9(Md22Calib)
  [Md56Calib] -> Subsystem/10(Md25Calib)
  [MD26Calib] -> Subsystem/11(Md26Calib)
  [Md21IsTargetPos] -> Subsystem1/20(Md21IsTargetPos)
  [Md56IsTargetPos] -> Subsystem1/22(Md25IsTargetPos)
  [Md26IsTargetPos] -> Subsystem1/23(Md26IsTargetPos)
  [Md22IsTargetPos] -> Subsystem1/21(Md22IsTargetPos)
  [Md21IsTargetPosAlready] -> Subsystem1/24(Md21IsTargetPosAlready)
  [Md22IsTargetPosAlready] -> Subsystem1/25(Md22IsTargetPosAlready)
  [Md56IsTargetPosAlready] -> Subsystem1/26(Md25IsTargetPosAlready)
  [Md26IsTargetPosAlready] -> Subsystem1/27(Md26IsTargetPosAlready)
  [Md21IsTargetPosZone] -> Subsystem1/28(Md21IsTargetPosZone)
  [Md22IsTargetPosZone] -> Subsystem1/29(Md22IsTargetPosZone)
  [Md56IsTargetPosZone] -> Subsystem1/30(Md25IsTargetPosZone)
  [Md26IsTargetPosZone] -> Subsystem1/31(Md26IsTargetPosZone)
  StNumFlg_Is4s_read/1 -> [Is4s], Subsystem1/32(StNumFlg_Is4s_read)
  KeSMSw4SVIPLMDFwdBkwdTrgtPosCalib_TrgtPosArray_read/1 -> [VIP4sLCalib]
  KeSMSw4sLegrstOpenLMdFwdBkwdTrgtPosCalib_TrgtPosArray_read/1 -> [LegrstOpenLCalib]
  KeSMSw4SLyingLMDFwdBkwdTrgtPosCalib_TrgtPosArray_read/1 -> [LyingLCalib]
  [LegrstOpenLCalib] -> Subsystem12/3(CalibArray)
  [LyingLCalib] -> Subsystem13/3(CalibArray)
  [VIP4sLCalib] -> Subsystem14/3(CalibArray)
  [Pos] -> Subsystem12/2(Pos)
  [PosV] -> Subsystem12/1(PosV)
  [PosDelta] -> Subsystem12/4(Delta)
  [PosTolr] -> Subsystem12/5(Tolr)
  [PosV] -> Subsystem13/1(PosV)
  [Pos] -> Subsystem13/2(Pos)
  [PosDelta] -> Subsystem13/4(Delta)
  [PosTolr] -> Subsystem13/5(Tolr)
  [PosTolr] -> Subsystem14/5(Tolr)
  [PosDelta] -> Subsystem14/4(Delta)
  [Pos] -> Subsystem14/2(Pos)
  [PosV] -> Subsystem14/1(PosV)
  Subsystem12/2(IsPosZone) -> [LgrstOpenLIsTargetPosZone]
  Subsystem12/3(IsPosAlready) -> [LgrstOpenLIsTargetPosAlready]
  Subsystem12/1(IsPos) -> [LgrstOpenLIsTargetPos]
  Subsystem13/1(IsPos) -> [LyLIsTargetPos]
  Subsystem13/2(IsPosZone) -> [LyLIsTargetPosZone]
  Subsystem13/3(IsPosAlready) -> [LyLIsTargetPosAlready]
  Subsystem14/1(IsPos) -> [VIP4sLIsTargetPos]
  Subsystem14/2(IsPosZone) -> [VIP4sLIsTargetPosZone]
  Subsystem14/3(IsPosAlready) -> [VIP4sLIsTargetPosAlready]
  [LegrstOpenLCalib] -> Subsystem/12(VIP4sLCalib)
  [LyingLCalib] -> ?
  [VIP4sLCalib] -> ?
  [Is4s] -> Subsystem/13(Is4s)
  [VIP4sLIsTargetPos] -> Subsystem1/33(VIP4sLIsTargetPos)
  [LyLIsTargetPos] -> Subsystem1/34(Ly4sLIsTargetPos)
  [LgrstOpenLIsTargetPos] -> Subsystem1/35(LgrstOpen4sLIsTargetPos)
  [VIP4sLIsTargetPosZone] -> Subsystem1/41(VIP4sLIsTargetPosZone)
  [VIP4sLIsTargetPosAlready] -> Subsystem1/36(VIP4sLIsTargetPosAlready)
  [LgrstOpenLIsTargetPosZone] -> Subsystem1/40(LgrstOpen4sLIsTargetPosZone)
  [LyLIsTargetPosZone] -> Subsystem1/39(Ly4sLIsTargetPosZone)
  [LgrstOpenLIsTargetPosAlready] -> Subsystem1/38(LgrstOpen4sLIsTargetPosAlready)
  [LyLIsTargetPosAlready] -> Subsystem1/37(Ly4sLIsTargetPosAlready)
  VIPLExitR2LFwdBkwdTrgtPosCalib_TrgtPosArray_read/1 -> [Md27Calib]
  [Pos] -> Subsystem15/2(Pos)
  Subsystem15/1(IsPos) -> [Md27IsTargetPos]
  [Md27Calib] -> Subsystem15/3(CalibArray)
  [PosTolr] -> Subsystem15/5(Tolr)
  [PosDelta] -> Subsystem15/4(Delta)
  Subsystem15/2(IsPosZone) -> [Md27IsTargetPosZone]
  [PosV] -> Subsystem15/1(PosV)
  [Md27Calib] -> Subsystem/14(Md27Calib)
  [Md27IsTargetPos] -> Subsystem1/42(Md27IsTargetPos)
  [Md27IsTargetPosAlready] -> Subsystem1/43(Md27IsTargetPosAlready)
  [Md27IsTargetPosZone] -> Subsystem1/44(Md27IsTargetPosZone)
  Subsystem15/3(IsPosAlready) -> [Md27IsTargetPosAlready]
  Md8R2LFwdBkwdTrgtPosCalib_TrgtPosArray_read/1 -> [Md8Calib]
  Subsystem16/3(IsPosAlready) -> [Md8IsTargetPosAlready]
  [PosV] -> Subsystem16/1(PosV)
  Subsystem16/2(IsPosZone) -> [Md8IsTargetPosZone]
  [PosDelta] -> Subsystem16/4(Delta)
  [PosTolr] -> Subsystem16/5(Tolr)
  [Md8Calib] -> Subsystem16/3(CalibArray)
  Subsystem16/1(IsPos) -> [Md8IsTargetPos]
  [Pos] -> Subsystem16/2(Pos)
  [Md8Calib] -> Subsystem/15(Md8Calib)
  StNumFlg_Is7s_read/1 -> Subsystem1/45(StNumFlg_Is7s_read)
  [Md8IsTargetPos] -> Subsystem1/46(Md8IsTargetPos)
  [Md8IsTargetPosZone] -> Subsystem1/48(Md8IsTargetPosZone)
  [Md8IsTargetPosAlready] -> Subsystem1/47(Md8IsTargetPosAlready)
  Bitwise Operator/1 -> Switch/1
  Switch/1 -> MdXXSecRwLtStFwdBkwdIsTargetPosAlready_Val_write/1
  Bitwise Operator1/1 -> Bitwise Operator/2
  Constant/1 -> Bitwise Operator1/1
  IfVeSMSbSecRwLtStCshnFrntUpwdDnwdMovConfig_Val_read/1 -> Switch/2
  Data Type Conversion2/1 -> Bitwise Operator/1, Switch/3
  Md56R2LFwdBkwdTrgtPosCalib_TrgtPosArray_read/1 -> [Md56Calib]
  [Pos] -> Subsystem17/2(Pos)
  [Md56Calib] -> Subsystem17/3(CalibArray)
  [PosTolr] -> Subsystem17/5(Tolr)
  [PosDelta] -> Subsystem17/4(Delta)
  [PosV] -> Subsystem17/1(PosV)
  Subsystem17/1(IsPos) -> [Md56IsTargetPos]
  Subsystem17/2(IsPosZone) -> [Md56IsTargetPosZone]
  Subsystem17/3(IsPosAlready) -> [Md56IsTargetPosAlready]
  Md62SecRwLtStFwdBkwdCalib_TrgtPosArray_read/1 -> [Md62Calib]
  Md61SecRwLtStFwdBkwdCalib_TrgtPosArray_read/1 -> [Md61Calib]
  Subsystem18/3(IsPosAlready) -> [Md61IsTargetPosAlready]
  Subsystem18/2(IsPosZone) -> [Md61IsTargetPosZone]
  Subsystem18/1(IsPos) -> [Md61IsTargetPos]
  [PosV] -> Subsystem18/1(PosV)
  [PosDelta] -> Subsystem18/4(Delta)
  [PosTolr] -> Subsystem18/5(Tolr)
  [Md61Calib] -> Subsystem18/3(CalibArray)
  [Pos] -> Subsystem18/2(Pos)
  [Pos] -> Subsystem19/2(Pos)
  [Md62Calib] -> Subsystem19/3(CalibArray)
  [PosTolr] -> Subsystem19/5(Tolr)
  [PosDelta] -> Subsystem19/4(Delta)
  [PosV] -> Subsystem19/1(PosV)
  Subsystem19/1(IsPos) -> [Md62IsTargetPos]
  Subsystem19/2(IsPosZone) -> [Md62IsTargetPosZone]
  Subsystem19/3(IsPosAlready) -> [Md62IsTargetPosAlready]
  [Md61Calib] -> Subsystem/16(Md61Calib)
  [Md62Calib] -> Subsystem/17(Md62Calib)
  [Md61IsTargetPos] -> Subsystem1/49(Md61IsTargetPos)
  [Md62IsTargetPos] -> Subsystem1/50(Md62IsTargetPos)
  [Md62IsTargetPosZone] -> Subsystem1/54(Md62IsTargetPosZone)
  [Md61IsTargetPosZone] -> Subsystem1/53(Md61IsTargetPosZone)
  [Md62IsTargetPosAlready] -> Subsystem1/52(Md62IsTargetPosAlready)
  [Md61IsTargetPosAlready] -> Subsystem1/51(Md61IsTargetPosAlready)

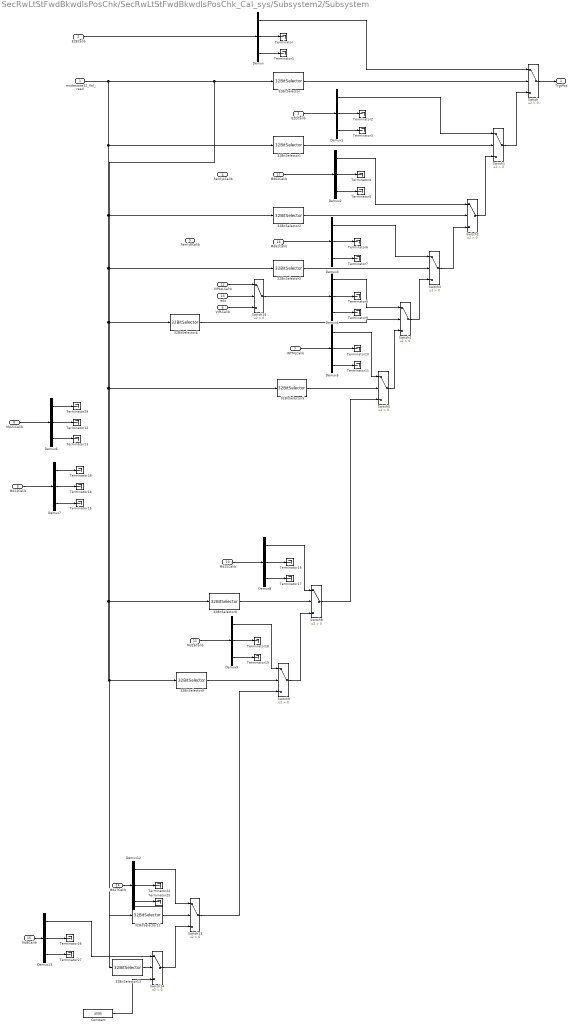
== system SecRwLtStFwdBkwdIsPosChk/SecRwLtStFwdBkwdIsPosChk_Cal_sys/Subsystem2/Subsystem ==
  modestate32_Val_read : Inport
  EZECalib : Inport  Port=2
  EZQCalib : Inport  Port=3
  FamlyLCalib : Inport  Port=4
  FamlyRCalib : Inport  Port=5
  VIPLCalib : Inport  Port=6
  INTMLCalib : Inport  Port=7
  Md21Calib : Inport  Port=8
  Md22Calib : Inport  Port=9
  Md25Calib : Inport  Port=10
  Md26Calib : Inport  Port=11
  VIP4sLCalib : Inport  Port=12
  Is4s : Inport  Port=13
  Md27Calib : Inport  Port=14
  Md8Calib : Inport  Port=15
  Md61Calib : Inport  Port=16
  Md62Calib : Inport  Port=17
  32BitSelector : StIsPosChkLib/32BitSelector  BitNum=0
  32BitSelector1 : StIsPosChkLib/32BitSelector  BitNum=3
  32BitSelector12 : StIsPosChkLib/32BitSelector  BitNum=26
  32BitSelector13 : StIsPosChkLib/32BitSelector  BitNum=7
  32BitSelector2 : StIsPosChkLib/32BitSelector  BitNum=6
  32BitSelector3 : StIsPosChkLib/32BitSelector  BitNum=5
  32BitSelector4 : StIsPosChkLib/32BitSelector  BitNum=9
  32BitSelector5 : StIsPosChkLib/32BitSelector  BitNum=4
  32BitSelector8 : StIsPosChkLib/32BitSelector  BitNum=24
  32BitSelector9 : StIsPosChkLib/32BitSelector  BitNum=25
  Constant : Constant  Value=4095  OutDataTypeStr=uint16
  Demux{,1..9,12..13} (12 alike) : Demux  Outputs=3
  Switch{,1..5,8..10,13..14} (11 alike) : Switch  Criteria=u2 > Threshold  SaturateOnIntegerOverflow=off  InputSameDT=off
  Terminator{,1..19,24..29} (26 alike) : Terminator
  TrgtPos : Outport  VectorParamsAs1DForOutWhenUnconnected=off
      settings: EnsureOutportIsVirtual=on
  wires:
  32BitSelector/1 -> Switch/2
  Demux/1 -> Switch/1
  Demux/3 -> Terminator1/1
  Demux/2 -> Terminator/1
  EZECalib/1 -> Demux/1
  EZQCalib/1 -> Demux1/1
  Demux1/2 -> Terminator2/1
  Demux1/3 -> Terminator3/1
  Demux1/1 -> Switch1/1
  Switch/1 -> TrgtPos/1
  Switch1/1 -> Switch/3
  32BitSelector1/1 -> Switch1/2
  Switch2/1 -> Switch1/3
  Switch3/1 -> Switch2/3
  Switch4/1 -> Switch3/3
  32BitSelector2/1 -> Switch2/2
  32BitSelector3/1 -> Switch3/2
  32BitSelector4/1 -> Switch4/2
  Demux2/1 -> Switch2/1
  Demux2/3 -> Terminator5/1
  Demux2/2 -> Terminator4/1
  Demux3/2 -> Terminator6/1
  Demux3/3 -> Terminator7/1
  Demux3/1 -> Switch3/1
  Demux4/1 -> Switch4/1
  Demux4/3 -> Terminator9/1
  Demux4/2 -> Terminator8/1
  INTMLCalib/1 -> Demux5/1
  Demux5/2 -> Terminator10/1
  Demux5/3 -> Terminator11/1
  Demux5/1 -> Switch5/1
  Switch5/1 -> Switch4/3
  32BitSelector5/1 -> Switch5/2
  Switch8/1 -> Switch5/3
  Demux6/3 -> Terminator13/1
  Demux6/2 -> Terminator12/1
  Md21Calib/1 -> Demux6/1
  Md22Calib/1 -> Demux7/1
  Demux7/2 -> Terminator14/1
  Demux7/3 -> Terminator15/1
  32BitSelector8/1 -> Switch8/2
  Demux8/1 -> Switch8/1
  Demux8/3 -> Terminator17/1
  Demux8/2 -> Terminator16/1
  Md25Calib/1 -> Demux8/1
  Md26Calib/1 -> Demux9/1
  Demux9/2 -> Terminator18/1
  Demux9/3 -> Terminator19/1
  Demux9/1 -> Switch9/1
  32BitSelector9/1 -> Switch9/2
  Switch9/1 -> Switch8/3
  Is4s/1 -> Switch10/2
  VIPLCalib/1 -> Switch10/3
  Switch10/1 -> Demux4/1
  VIP4sLCalib/1 -> Switch10/1
  Switch13/1 -> Switch9/3
  Demux12/1 -> Switch13/1
  Demux12/3 -> Terminator25/1
  Demux12/2 -> Terminator24/1
  Md27Calib/1 -> Demux12/1
  32BitSelector12/1 -> Switch13/2
  Switch14/1 -> Switch13/3
  Constant/1 -> Switch14/3
  Md8Calib/1 -> Demux13/1
  Demux13/2 -> Terminator26/1
  Demux13/3 -> Terminator27/1
  Demux13/1 -> Switch14/1
  32BitSelector13/1 -> Switch14/2
  modestate32_Val_read/1 -> 32BitSelector13/1, 32BitSelector/1, 32BitSelector1/1, 32BitSelector2/1, 32BitSelector3/1, 32BitSelector4/1, 32BitSelector5/1, 32BitSelector8/1, 32BitSelector12/1, 32BitSelector9/1
  Demux7/1 -> Terminator28/1
  Demux6/1 -> Terminator29/1
  Md61Calib/1 -> Demux3/1
  Md62Calib/1 -> Demux2/1
